simulink model "mode_selection_unit_test"  (R2016b)
settings: Solver=VariableStepAuto  StartTime=0.0  StopTime=10.0  RelTol=1e-3
libraries: mode_selection x1
settings Model: Creator=taylorreynolds  LastModifiedBy=taylorreynolds

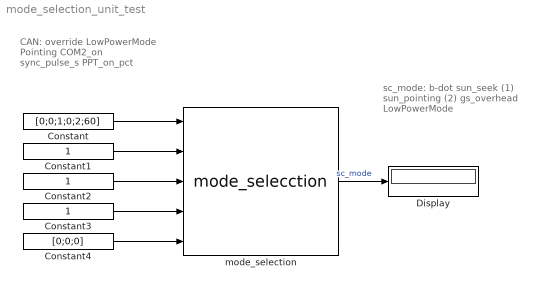
== system mode_selection_unit_test ==
  note: sc_mode:
      | b-dot
      | sun_seek
      |
      | (1) sun_pointing
      | (2) gs_overhead
      | LowPowerMode
  note: CAN:
      | override
      | LowPowerMode
      | Pointing
      | COM2_on
      | sync_pulse_s
      | PPT_on_pct
  Constant : Constant  Value=[0;0;1;0;2;60]  OutDataTypeStr=int8
  Constant1 : Constant
  Constant2 : Constant
  Constant3 : Constant
  Constant4 : Constant  Value=[0;0;0]
  Display : Display
  mode_selection : mode_selection/mode_selecction
  wires:
  mode_selection/1 -> Display/1  "sc_mode"
  Constant2/1 -> mode_selection/3
  Constant3/1 -> mode_selection/4
  Constant4/1 -> mode_selection/5
  Constant/1 -> mode_selection/1
  Constant1/1 -> mode_selection/2
